simulink model "LQRController"  (R2024b)
settings: Solver=ode45  StartTime=0.0  StopTime=10  MaxStep=0.001  RelTol=1e-3
values from neighbouring files (symbols this model uses):
  A = [0 1 0 0 0 0 0 0 ... (first row only)    [LQR.m]
  A_inverse = inv(alloc_matrix)    [controlalloc.m]
  B = [0 0 0 0 ... (first row only)    [LQR.m]
undefined symbols (not defined in the file or in its folder): Q, R
settings Model: Creator=shree  LastModifiedBy=shree
settings SolverCC: MaxConsecutiveMinStep=5
settings RTWCC: GenerateReport=on  LaunchReport=on

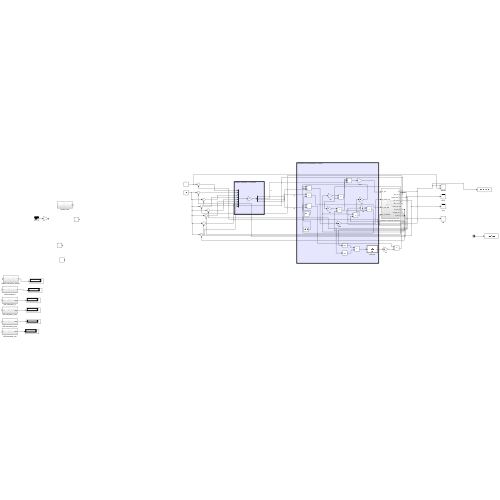
[thumbnail: Simulink's stored preview of the top-level diagram]
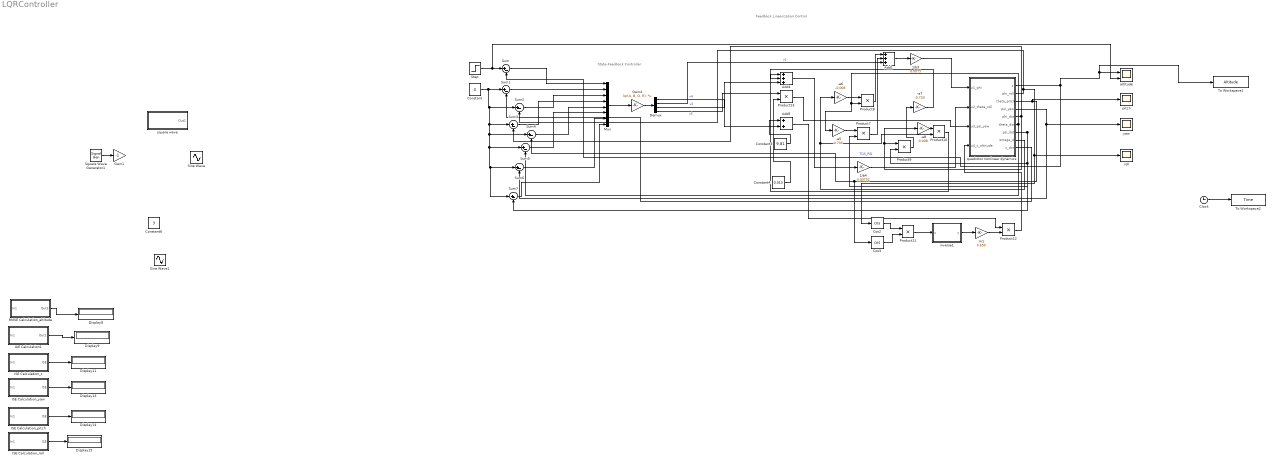
== system LQRController ==
  note: Feedback Linearization Control
  note: State-Feedback Controller
  -a5 : Gain  Gain=0.733
  -a6 : Gain  Gain=-0.008
  -a7 : Gain  Gain=-0.733
  -a8 : Gain  Gain=0.008
  1/b3 : Gain  Gain=0.0075
  1/b4 : Gain  Gain=0.00752
  Add1 : Sum  Inputs=+++
  Add4 : Sum  Inputs=+++
  Add5 : Sum
  Clock : Clock
  Constant : Constant  Value=0
  Constant3 : Constant  Value=9.81
  Constant4 : Constant  Value=0.013
  Constant6 : Constant  Value=3
  Cos2 : Trigonometry  Operator=cos
  Cos3 : Trigonometry  Operator=cos
  Demux : Demux
  Display{8..9,11,13..15} (6 alike) : Display
  Gain1 : Gain  Gain=-1
  Gain4 : Gain  Gain=lqr(A, B, Q, R);  Multiplication=Matrix(K*u)
  IAE Calculation1 : Subsystem
  ISE Calculation_pitch : Subsystem
  ISE Calculation_roll : Subsystem
  ISE Calculation_yaw : Subsystem
  ISE Calculation_z : Subsystem
  Mux : Mux  Inputs=8
  Product{7..13} (7 alike) : Product
  RMSE Calculation_altitude : Subsystem
  Sine Wave : Sin  Amplitude=3  Frequency=3  SampleTime=0
  Sine Wave1 : Sin  Amplitude=3  SampleTime=0
  Square Wave Generator1 : SignalGenerator  WaveForm=square  Amplitude=3
  Step : Step  Time=0  After=-1  SampleTime=0
  Sum{,1..7} (8 alike) : Sum  Inputs=|+-
  To Workspace1 : ToWorkspace  VariableName=Altitude  SaveFormat=Timeseries  SampleTime=-1
  To Workspace2 : ToWorkspace  VariableName=Time  SaveFormat=Timeseries  SampleTime=-1
  altitude : Scope  NumInputPorts=2
  inverse1 : MATLAB Function  TreatAsAtomicUnit=on
  m1 : Gain  Gain=0.650
  pitch : Scope
  quadrotor nonlinear dynamics : Subsystem
  roll : Scope
  square wave : Subsystem
  yaw : Scope
  wires:
  Product7/1 -> Add1/2
  RMSE Calculation_altitude/1(Out1) -> Display8/1
  Product9/1 -> -a7/1
  quadrotor nonlinear dynamics/7(psi_dot) -> Sum7/2, Product9/2, Product7/2
  -a6/1 -> Product8/1
  quadrotor nonlinear dynamics/5(phi_dot) -> Sum3/2, -a8/1, Product9/1
  Cos3/1 -> Product11/2
  Product10/1 -> Add4/1
  -a7/1 -> Add4/2
  Demux/4 -> Product13/1  "v3"
  ISE Calculation_pitch/1(ISE) -> Display14/1
  Product12/1 -> quadrotor nonlinear dynamics/4(u4_z_altitude)
  Demux/2 -> Add1/3  "v1"
  Demux/3 -> Add4/3  "v2"
  Constant3/1 -> Add5/1
  ISE Calculation_z/1(ISE) -> Display11/1
  m1/1 -> Product12/2
  -a8/1 -> Product10/1
  Cos2/1 -> Product11/1
  Add4/1 -> 1/b4/1
  Product11/1 -> inverse1/1(u)
  Add1/1 -> 1/b3/1
  ISE Calculation_yaw/1(ISE) -> Display13/1
  Product8/1 -> Add1/1
  Add5/1 -> Product12/1
  Constant4/1 -> Product13/2
  -a5/1 -> Product7/1
  inverse1/1(y) -> m1/1
  1/b4/1 -> quadrotor nonlinear dynamics/2(u2_theta_roll)
  quadrotor nonlinear dynamics/6(theta_dot) -> Sum5/2, -a5/1, Product8/2
  ISE Calculation_roll/1(ISE) -> Display15/1
  quadrotor nonlinear dynamics/2(phi_roll) -> Sum2/2, roll/1, Cos2/1
  Square Wave Generator1/1 -> Gain1/1
  IAE Calculation1/1(Out1) -> Display9/1
  quadrotor nonlinear dynamics/8(omega_d) -> Product10/2, -a6/1
  Demux/1 -> Add5/2  "v4"
  quadrotor nonlinear dynamics/3(theta_pitch) -> Sum4/2, Cos3/1, pitch/1
  1/b3/1 -> quadrotor nonlinear dynamics/1(u1_phi)
  Product13/1 -> quadrotor nonlinear dynamics/3(u3_psi_yaw)
  quadrotor nonlinear dynamics/1(z) -> Sum/2, To Workspace1/1, altitude/1  "TD3_PID"
  quadrotor nonlinear dynamics/4(psi_yaw) -> Sum6/2, yaw/1
  quadrotor nonlinear dynamics/9(z_dot) -> Sum1/2
  Step/1 -> altitude/2, Sum/1
  Constant/1 -> Sum7/1, Sum6/1, Sum5/1, Sum4/1, Sum3/1, Sum2/1, Sum1/1
  Mux/1 -> Gain4/1
  Sum/1 -> Mux/1
  Sum1/1 -> Mux/2
  Sum2/1 -> Mux/3
  Sum3/1 -> Mux/4
  Sum4/1 -> Mux/5
  Sum5/1 -> Mux/6
  Sum6/1 -> Mux/7
  Sum7/1 -> Mux/8
  Gain4/1 -> Demux/1
  Clock/1 -> To Workspace2/1

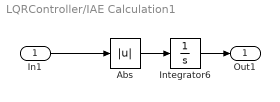
== system LQRController/IAE Calculation1 ==
  In1 : Inport
  Abs : Abs  SaturateOnIntegerOverflow=off
  Integrator6 : Integrator
  Out1 : Outport
  wires:
  Abs/1 -> Integrator6/1
  Integrator6/1 -> Out1/1
  In1/1 -> Abs/1

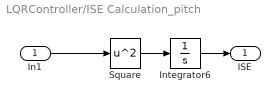
== system LQRController/ISE Calculation_pitch ==
  In1 : Inport
  Integrator6 : Integrator
  Square : Math  Operator=square
  ISE : Outport
  wires:
  Square/1 -> Integrator6/1
  Integrator6/1 -> ISE/1
  In1/1 -> Square/1

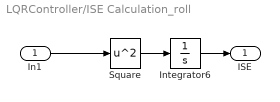
== system LQRController/ISE Calculation_roll ==
  In1 : Inport
  Integrator6 : Integrator
  Square : Math  Operator=square
  ISE : Outport
  wires:
  Square/1 -> Integrator6/1
  Integrator6/1 -> ISE/1
  In1/1 -> Square/1

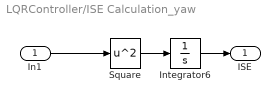
== system LQRController/ISE Calculation_yaw ==
  In1 : Inport
  Integrator6 : Integrator
  Square : Math  Operator=square
  ISE : Outport
  wires:
  Square/1 -> Integrator6/1
  Integrator6/1 -> ISE/1
  In1/1 -> Square/1

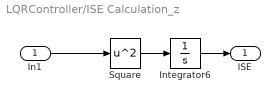
== system LQRController/ISE Calculation_z ==
  In1 : Inport
  Integrator6 : Integrator
  Square : Math  Operator=square
  ISE : Outport
  wires:
  Square/1 -> Integrator6/1
  Integrator6/1 -> ISE/1
  In1/1 -> Square/1

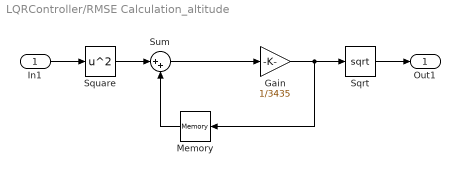
== system LQRController/RMSE Calculation_altitude ==
  In1 : Inport
  Gain : Gain  Gain=1/3435
  Memory : Memory
  Sqrt : Sqrt
  Square : Math  Operator=square
  Sum : Sum  Inputs=|++
  Out1 : Outport
  wires:
  In1/1 -> Square/1
  Square/1 -> Sum/1
  Memory/1 -> Sum/2
  Sum/1 -> Gain/1
  Gain/1 -> Sqrt/1, Memory/1
  Sqrt/1 -> Out1/1

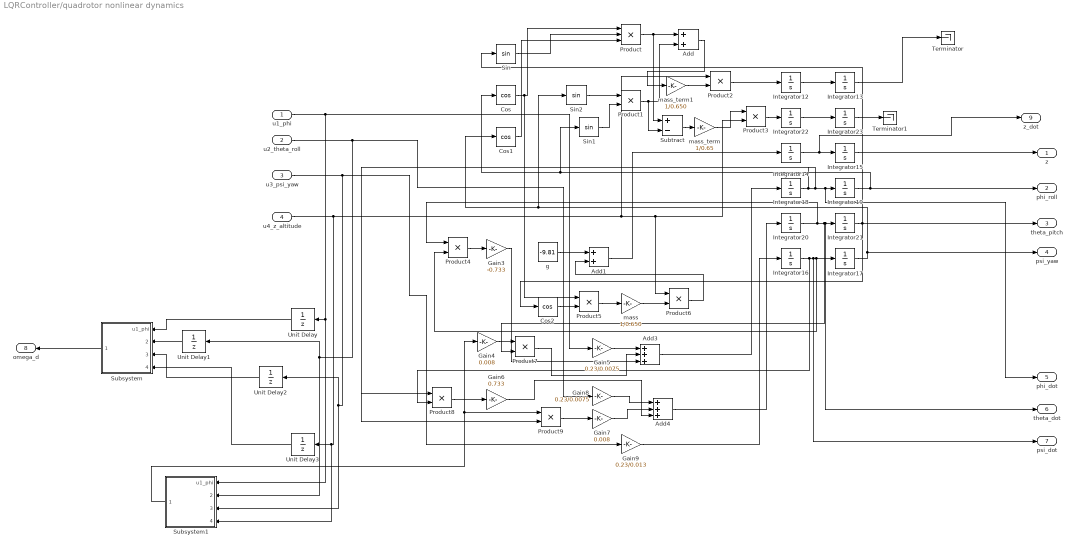
== system LQRController/quadrotor nonlinear dynamics ==
  u1_phi : Inport
  u2_theta_roll : Inport  Port=2
  u3_psi_yaw : Inport  Port=3
  u4_z_altitude : Inport  Port=4
  Add : Sum
  Add1 : Sum
  Add3 : Sum  Inputs=+++
  Add4 : Sum  Inputs=+++
  Cos : Trigonometry  Operator=cos
  Cos1 : Trigonometry  Operator=cos
  Cos2 : Trigonometry  Operator=cos
  Gain3 : Gain  Gain=-0.733
  Gain4 : Gain  Gain=0.008
  Gain5 : Gain  Gain=0.23/0.0075
  Gain6 : Gain  Gain=0.733
  Gain7 : Gain  Gain=0.008
  Gain8 : Gain  Gain=0.23/0.0075
  Gain9 : Gain  Gain=0.23/0.013
  Integrator{12..15,18,20,22..23} (8 alike) : Integrator
  Integrator{16..17,19,21} (4 alike) : Integrator  LowerSaturationLimit=0
  Product : Product  Inputs=3
  Product{1..9} (9 alike) : Product
  Sin : Trigonometry
  Sin1 : Trigonometry
  Sin2 : Trigonometry
  Subsystem : Subsystem
  Subsystem1 : Subsystem
  Subtract : Sum  Inputs=+-
  Terminator : Terminator
  Terminator1 : Terminator
  Unit Delay{,1..3} (4 alike) : UnitDelay  SampleTime=-1  HasFrameUpgradeWarning=on
  g : Constant  Value=-9.81
  mass : Gain  Gain=1/0.650
  mass_term : Gain  Gain=1/0.65
  mass_term1 : Gain  Gain=1/0.650
  z : Outport
  phi_roll : Outport  Port=2
  theta_pitch : Outport  Port=3
  psi_yaw : Outport  Port=4
  phi_dot : Outport  Port=5
  theta_dot : Outport  Port=6
  psi_dot : Outport  Port=7
  omega_d : Outport  Port=8
  z_dot : Outport  Port=9
  wires:
  Gain9/1 -> Integrator16/1
  Product9/1 -> Gain7/1
  Gain6/1 -> Add4/3
  Add3/1 -> Integrator18/1
  Add4/1 -> Integrator20/1
  Gain7/1 -> Add4/2
  Gain4/1 -> Product7/1
  Product7/1 -> Add3/2
  Product1/1 -> Subtract/2, Add/2
  g/1 -> Add1/1
  mass_term/1 -> Product3/1
  Integrator18/1 -> Product9/2, Product8/1, phi_dot/1, Integrator19/1
  mass/1 -> Product6/2
  Gain8/1 -> Add4/1
  mass_term1/1 -> Product2/2
  Gain5/1 -> Add3/1
  Product5/1 -> mass/1
  Integrator12/1 -> Integrator13/1
  Product/1 -> Subtract/1, Add/1
  Product2/1 -> Integrator12/1
  Integrator15/1 -> z/1
  Integrator22/1 -> Integrator23/1
  Add1/1 -> Integrator14/1
  Integrator14/1 -> z_dot/1, Integrator15/1
  Cos1/1 -> Product/3
  Cos/1 -> Product5/1, Product/1
  Integrator17/1 -> Sin2/1, Cos1/1, psi_yaw/1
  Sin1/1 -> Product1/2
  Integrator20/1 -> Integrator21/1, theta_dot/1, Product7/2, Product4/1
  Integrator16/1 -> Product8/2, Product4/2, Integrator17/1, psi_dot/1
  Integrator21/1 -> theta_pitch/1, Cos2/1, Sin/1
  Add/1 -> mass_term1/1
  Product4/1 -> Gain3/1
  Product6/1 -> Add1/2
  Sin2/1 -> Product1/1
  Product8/1 -> Gain6/1
  Sin/1 -> Product/2
  Cos2/1 -> Product5/2
  Product3/1 -> Integrator22/1
  Subtract/1 -> mass_term/1
  Gain3/1 -> Add3/3
  Integrator19/1 -> Sin1/1, Cos/1, phi_roll/1
  u1_phi/1 -> Subsystem1/1(u1_phi), Unit Delay/1, Gain5/1
  u4_z_altitude/1 -> Product3/2, Product6/1, Product2/1, Subsystem1/4(u4_z_altitude), Unit Delay3/1
  u3_psi_yaw/1 -> Subsystem1/3(u3_psi_yaw), Unit Delay2/1, Gain9/1
  u2_theta_roll/1 -> Subsystem1/2(u2_theta_roll), Unit Delay1/1, Gain8/1
  Unit Delay/1 -> Subsystem/1(u1_phi)
  Unit Delay1/1 -> Subsystem/2(u2_theta_roll)
  Unit Delay2/1 -> Subsystem/3(u3_psi_yaw)
  Unit Delay3/1 -> Subsystem/4(u4_z_altitude)
  Integrator13/1 -> Terminator/1
  Integrator23/1 -> Terminator1/1
  Subsystem/1(omega_d) -> omega_d/1
  Subsystem1/1(omega_d) -> Product9/1, Gain4/1

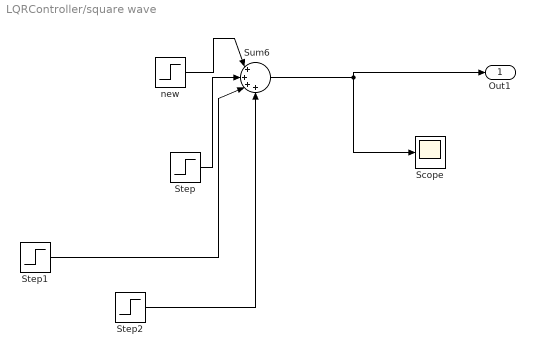
== system LQRController/square wave ==
  Scope : Scope
  Step : Step  Time=4  SampleTime=0
  Step1 : Step  Time=8  After=-1  SampleTime=0
  Step2 : Step  Time=10  After=-1  SampleTime=0
  Sum6 : Sum  Inputs=|++++
  new : Step  Time=2  SampleTime=0.1
  Out1 : Outport
  wires:
  Sum6/1 -> Out1/1, Scope/1
  Step/1 -> Sum6/2
  new/1 -> Sum6/1
  Step1/1 -> Sum6/3
  Step2/1 -> Sum6/4

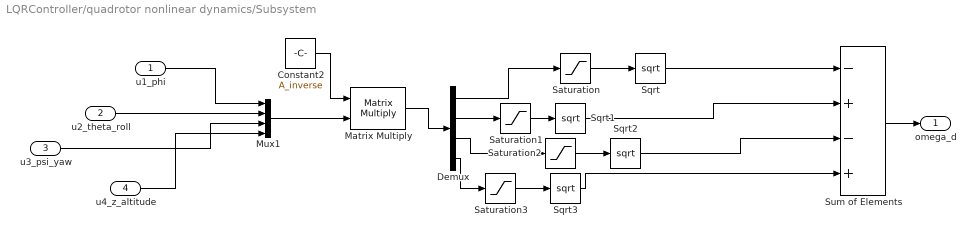
== system LQRController/quadrotor nonlinear dynamics/Subsystem ==
  u1_phi : Inport
  u2_theta_roll : Inport  Port=2
  u3_psi_yaw : Inport  Port=3
  u4_z_altitude : Inport  Port=4
  Constant2 : Constant  Value=A_inverse
  Demux : Demux
  Matrix Multiply : Product  Multiplication=Matrix(*)
  Mux1 : Mux
  Saturation{,1..3} (4 alike) : Saturate  UpperLimit=490000  LowerLimit=0
  Sqrt{,1..3} (4 alike) : Sqrt
  Sum of Elements : Sum  Inputs=-+-+
  omega_d : Outport
  wires:
  Mux1/1 -> Matrix Multiply/2
  Saturation2/1 -> Sqrt2/1
  Demux/4 -> Saturation3/1
  u1_phi/1 -> Mux1/1
  Sqrt1/1 -> Sum of Elements/2
  Sqrt/1 -> Sum of Elements/1
  Saturation1/1 -> Sqrt1/1
  Constant2/1 -> Matrix Multiply/1
  Saturation/1 -> Sqrt/1
  Matrix Multiply/1 -> Demux/1
  Saturation3/1 -> Sqrt3/1
  Demux/2 -> Saturation1/1
  Demux/1 -> Saturation/1
  Demux/3 -> Saturation2/1
  Sqrt2/1 -> Sum of Elements/3
  u3_psi_yaw/1 -> Mux1/3
  u2_theta_roll/1 -> Mux1/2
  Sqrt3/1 -> Sum of Elements/4
  u4_z_altitude/1 -> Mux1/4
  Sum of Elements/1 -> omega_d/1

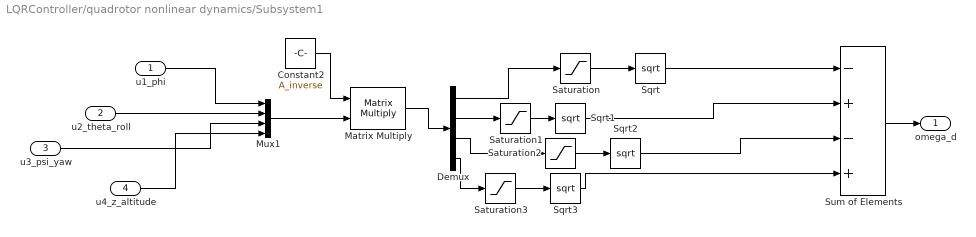
== system LQRController/quadrotor nonlinear dynamics/Subsystem1 ==
  u1_phi : Inport
  u2_theta_roll : Inport  Port=2
  u3_psi_yaw : Inport  Port=3
  u4_z_altitude : Inport  Port=4
  Constant2 : Constant  Value=A_inverse
  Demux : Demux
  Matrix Multiply : Product  Multiplication=Matrix(*)
  Mux1 : Mux
  Saturation{,1..3} (4 alike) : Saturate  UpperLimit=490000  LowerLimit=0
  Sqrt{,1..3} (4 alike) : Sqrt
  Sum of Elements : Sum  Inputs=-+-+
  omega_d : Outport
  wires:
  Mux1/1 -> Matrix Multiply/2
  Saturation2/1 -> Sqrt2/1
  Demux/4 -> Saturation3/1
  u1_phi/1 -> Mux1/1
  Sqrt1/1 -> Sum of Elements/2
  Sqrt/1 -> Sum of Elements/1
  Saturation1/1 -> Sqrt1/1
  Constant2/1 -> Matrix Multiply/1
  Saturation/1 -> Sqrt/1
  Matrix Multiply/1 -> Demux/1
  Saturation3/1 -> Sqrt3/1
  Demux/2 -> Saturation1/1
  Demux/1 -> Saturation/1
  Demux/3 -> Saturation2/1
  Sqrt2/1 -> Sum of Elements/3
  u3_psi_yaw/1 -> Mux1/3
  u2_theta_roll/1 -> Mux1/2
  Sqrt3/1 -> Sum of Elements/4
  u4_z_altitude/1 -> Mux1/4
  Sum of Elements/1 -> omega_d/1

== matlab function LQRController/inverse1 ==
  data: u input; y output
function y = fcn(u)

y = 1/u;
